simulink model "MKRCanPruebaMotores"  (R2023b)
settings: Solver=VariableStepAuto  StartTime=0.0  StopTime=10.0  RelTol=1e-3
model workspace (MAT data in the model file):
  Can_ID = 0
undefined symbols (not defined in the file): canChannel
libraries: canmsglib x3, arduinolib x2, canlib x1
settings Model: Creator=Antonio  LastModifiedBy=Antonio

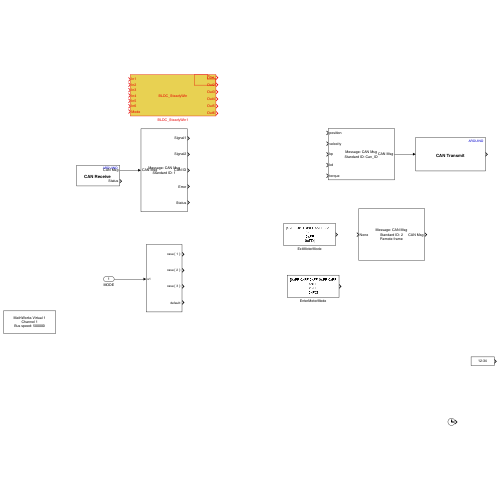
[thumbnail: Simulink's stored preview of the top-level diagram]
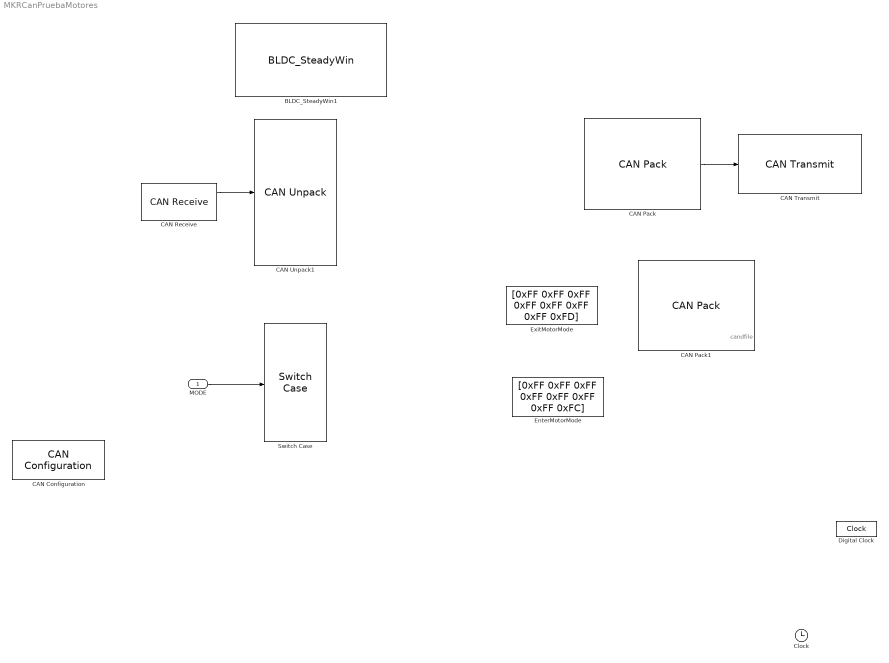
== system MKRCanPruebaMotores ==
  note: candfile
  MODE : Inport
  BLDC_SteadyWin1 : S-Function  InitFcn=try, set_param(gcb,'FunctionName','BLDC_SteadyWin'), end  FunctionName=BLDC_SteadyWin  SFunctionModules=BLDC_SteadyWinPack_wrapper.cpp  SFunctionDeploymentMode=off  EnableBusSupport=off  mask(S-Function Builder){}
      mask help: Simulink:masks:SFunctionBuilder_MD
      mask init:
      | val = [[.9  0.75 0.75 1 1 .9 .9 1]',[1 1 0.75 0.75 .9 .9 1 .9]'];try , sys = get_param(gcb,'SfunBuilderFcnName');if isempty(sys), sys = get_param(gcb,'FunctionName'); end,catch, sys = get_param(gcb,'FunctionName'); end
      settings: CopyFcn=set_param(gcbh,'LinkStatus','none')  PreSaveFcn=try, set_param(gcb,'FunctionName','BLDC_SteadyWin'), end  OpenFcn=sfunctionwizard(gcbh)
      mask Display:
      | plot(val(:,1),val(:,2))
      | disp(sys)
      | port_label('input',1,'In1')
      | port_label('input',2,'In2')
      | port_label('input',3,'In3')
      | port_label('input',4,'In4')
      | port_label('input',5,'In5')
      | port_label('input',6,'In6')
      | port_label('input',7,'Mode')
      | port_label('output',1,'Out1')
      | port_label('output',2,'Out2')
      | port_label('output',3,'Out3')
      | port_label('output',4,'Out4')
      | port_label('output',5,'Out5')
      | port_label('output',6,'Out6')
  CAN Configuration : canlib/CAN Configuration  BlockHandle=8729.0001  Device=MathWorks Virtual 1 (Channel 1)  DeviceMenu=MathWorks Virtual 1 (Channel 1)  ObjConstructor=canChannel('MathWorks', 'Virtual 1', 1)  BusSpeed=500000  EnableBitParameters=off  AckMode=Normal
  CAN Pack : canmsglib/CAN Pack  MsgList=(none)  MsgName=CAN Msg  MsgIDType=Standard (11-bit identifier)  MsgIdentifier=Can_ID  MsgLength=8  Remote=off  ApplyMinMax=off  BusOutput=off  SignalInfo={ 'position', '8', '16', 'BE', 'signed', 'Standard', '0', '1', '-95.5', '-95.5', '95.5'; 'velocity', '28', '12', 'BE', 'signed', 'Standard', '0', '1', '-45', '-45', '45'; 'kp', '32', '12', 'BE', 'unsigned', 'Standard', '0', '1', '0', '0', '500'; 'kd', '52', '12', 'BE', 'unsigned', 'Standard', '0', '1', '0', '0', '5'; 'torque', '56', '12', 'BE', 'signed', 'Standard', '0', '1', '-18', '-18', '18' }
      settings: LibrarySourceBlock=embeddedtargetslib/Host Communication/CAN Pack  DataFormat=manually specified signals
  CAN Pack1 : canmsglib/CAN Pack  MsgList=(none)  MsgName=CAN Msg  MsgIDType=Standard (11-bit identifier)  MsgIdentifier=2  MsgLength=8  Remote=on  ApplyMinMax=off  BusOutput=on  SignalInfo={ 'position', '8', '16', 'BE', 'signed', 'Standard', '0', '1', '-95.5', '-95.5', '95.5'; 'velocity', '28', '12', 'BE', 'signed', 'Standard', '0', '1', '-45', '-45', '45'; 'kp', '32', '12', 'BE', 'unsigned', 'Standard', '0', '1', '0', '0', '500'; 'kd', '52', '12', 'BE', 'unsigned', 'Standard', '0', '1', '0', '0', '5'; 'torque', '56', '12', 'BE', 'signed', 'Standard', '0', '1', '-18', '-18', '18' }
      settings: LibrarySourceBlock=embeddedtargetslib/Host Communication/CAN Pack  DataFormat=raw data
  CAN Receive : arduinolib/CAN Receive  outputDataType=CAN Msg  identifierType=Standard (11-bit identifier)  messageId=100  msgLength=8  SampleTime=0.1  outputError=off  outputRemote=off
  CAN Transmit : arduinolib/CAN Transmit  inputDataType=CAN Msg  BlockingMode_=on  BlockTimeout_=1  outputStatus=on  identifierType=Standard (11-bit identifier)  messageId=100  msgLength=8  remoteFrame=off
  CAN Unpack1 : canmsglib/CAN Unpack  MsgList=(none)  MsgName=CAN Msg  MsgIDType=Standard (11-bit identifier)  MsgIdentifier=1  MsgLength=8  SignalInfo={ 'Signal1', '0', '8', 'LE', 'signed', 'Standard', '0', '1', '0', '-Inf', 'Inf'; 'Signal2', '9', '8', 'LE', 'signed', 'Standard', '0', '1', '0', '-Inf', 'Inf' }  IDPort=on  TimestampPort=off  ErrorPort=on  RemotePort=off  LengthPort=off  StatusPort=on  ApplyMinMax=off
      settings: LibrarySourceBlock=embeddedtargetslib/Host Communication/CAN Unpack
  Clock : Clock
  Digital Clock : DigitalClock
  EnterMotorMode : Constant  Value=|  OutDataTypeStr=uint8
      | [0xFF 0xFF 0xFF 0xFF 0xFF
      | 0xFF
      | 0xFF
      | 0xFC]
  ExitMotorMode : Constant  Value=|  OutDataTypeStr=uint8
      | [0xFF 0xFF 0xFF 0xFF 0xFF
      | 0xFF
      | 0xFF
      | 0xFD]
  Switch Case : SwitchCase  CaseConditions={1 2 3}
  wires:
  CAN Receive/1 -> CAN Unpack1/1
  MODE/1 -> Switch Case/1
  CAN Pack/1 -> CAN Transmit/1
